simulink model "Lab3Model"  (R2021a)
settings: Solver=VariableStepAuto  StartTime=0.0  StopTime=10.0  MaxStep=10e-4  RelTol=1e-3
settings Model: Creator=Luka  LastModifiedBy=Luka

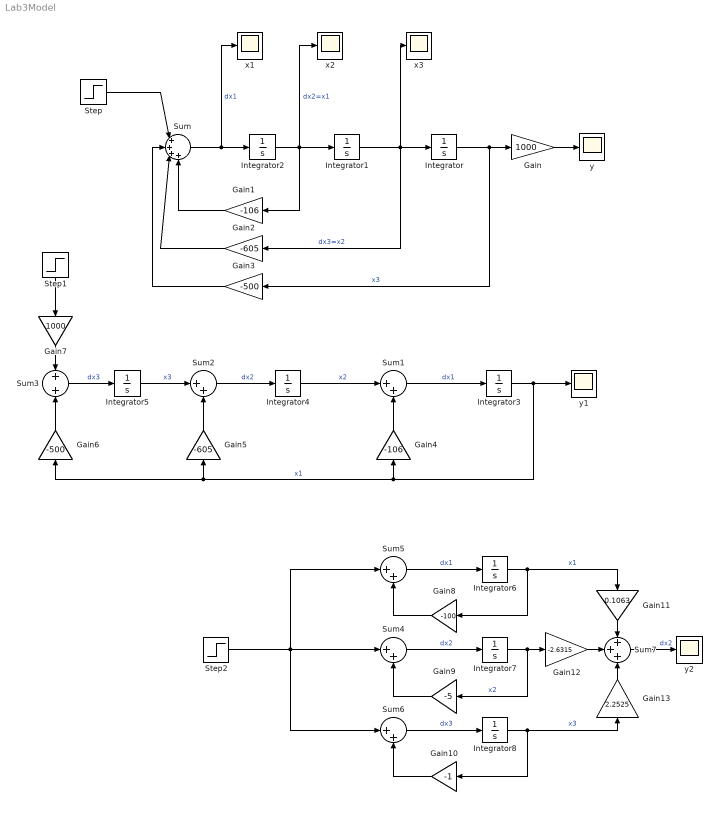
== system Lab3Model ==
  Gain : Gain  Gain=1000
  Gain1 : Gain  Gain=-106
  Gain10 : Gain  Gain=-1
  Gain11 : Gain  Gain=0.1063
  Gain12 : Gain  Gain=-2.6315
  Gain13 : Gain  Gain=2.2525
  Gain2 : Gain  Gain=-605
  Gain3 : Gain  Gain=-500
  Gain4 : Gain  Gain=-106
  Gain5 : Gain  Gain=-605
  Gain6 : Gain  Gain=-500
  Gain7 : Gain  Gain=1000
  Gain8 : Gain  Gain=-100
  Gain9 : Gain  Gain=-5
  Integrator{,1..8} (9 alike) : Integrator
  Step : Step  Time=0  SampleTime=0
  Step1 : Step  Time=0  SampleTime=0
  Step2 : Step  Time=0  SampleTime=0
  Sum : Sum  Inputs=|++++
  Sum{1..2,4..6} (5 alike) : Sum  Inputs=|++
  Sum3 : Sum
  Sum7 : Sum  Inputs=+++
  x1 : Scope
  x2 : Scope
  x3 : Scope
  y : Scope
  y1 : Scope
  y2 : Scope
  wires:
  Gain/1 -> y/1
  Integrator/1 -> Gain3/1, Gain/1  "x3"
  Integrator1/1 -> Gain2/1, x3/1, Integrator/1  "dx3=x2"
  Integrator2/1 -> x2/1, Gain1/1, Integrator1/1  "dx2=x1"
  Sum/1 -> x1/1, Integrator2/1  "dx1"
  Gain1/1 -> Sum/4
  Gain2/1 -> Sum/3
  Gain3/1 -> Sum/2
  Step/1 -> Sum/1
  Integrator3/1 -> Gain6/1, Gain5/1, Gain4/1, y1/1  "x1"
  Sum1/1 -> Integrator3/1  "dx1"
  Gain4/1 -> Sum1/2
  Integrator4/1 -> Sum1/1  "x2"
  Sum2/1 -> Integrator4/1  "dx2"
  Gain5/1 -> Sum2/2
  Integrator5/1 -> Sum2/1  "x3"
  Gain6/1 -> Sum3/2
  Sum3/1 -> Integrator5/1  "dx3"
  Gain7/1 -> Sum3/1
  Step1/1 -> Gain7/1
  Integrator6/1 -> Gain11/1, Gain8/1  "x1"
  Integrator7/1 -> Gain12/1, Gain9/1  "x2"
  Integrator8/1 -> Gain13/1, Gain10/1  "x3"
  Sum6/1 -> Integrator8/1  "dx3"
  Sum4/1 -> Integrator7/1  "dx2"
  Sum5/1 -> Integrator6/1  "dx1"
  Gain10/1 -> Sum6/2
  Gain9/1 -> Sum4/2
  Gain8/1 -> Sum5/2
  Step2/1 -> Sum6/1, Sum5/1, Sum4/1
  Sum7/1 -> y2/1  "dx2"
  Gain11/1 -> Sum7/1
  Gain12/1 -> Sum7/2
  Gain13/1 -> Sum7/3
